simulink model "TST_PTODi_TrqLeadCoord"  (R2016b)
settings: Solver=FixedStepDiscrete  StartTime=0.0  StopTime=simTime  FixedStep=sampleTime  RelTol=1e-3
values from neighbouring files (symbols this model uses):
  testCase = 1    [initTST_PTODi_TrqLeadCoord_001.m]
libraries: simulink x4, UnitTest_Lib x2
settings Model: Creator=zhengjinyan  LastModifiedBy=zhengjinyan
settings DebuggingCC: SignalRangeChecking=error

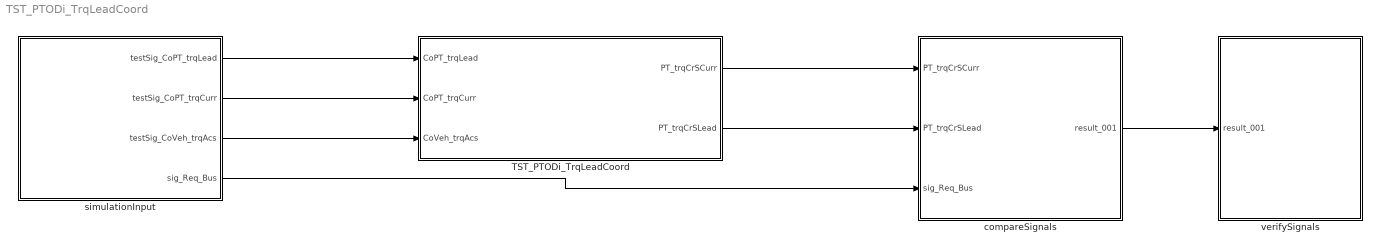
== system TST_PTODi_TrqLeadCoord ==
  TST_PTODi_TrqLeadCoord : Subsystem
  compareSignals : Subsystem
  simulationInput : Subsystem
  verifySignals : Subsystem
  wires:
  simulationInput/1(testSig_CoPT_trqLead) -> TST_PTODi_TrqLeadCoord/1(CoPT_trqLead)
  simulationInput/2(testSig_CoPT_trqCurr) -> TST_PTODi_TrqLeadCoord/2(CoPT_trqCurr)
  simulationInput/3(testSig_CoVeh_trqAcs) -> TST_PTODi_TrqLeadCoord/3(CoVeh_trqAcs)
  TST_PTODi_TrqLeadCoord/1(PT_trqCrSCurr) -> compareSignals/1(PT_trqCrSCurr)
  TST_PTODi_TrqLeadCoord/2(PT_trqCrSLead) -> compareSignals/2(PT_trqCrSLead)
  simulationInput/4(sig_Req_Bus) -> compareSignals/3(sig_Req_Bus)
  compareSignals/1(result_001) -> verifySignals/1(result_001)

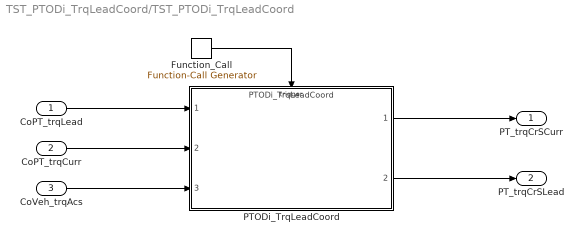
== system TST_PTODi_TrqLeadCoord/TST_PTODi_TrqLeadCoord ==
  CoPT_trqLead : Inport
  CoPT_trqCurr : Inport  Port=2
  CoVeh_trqAcs : Inport  Port=3
  Function_Call : simulink/Ports & Subsystems/Function-Call Generator  sample_time=sampleTime  numberOfIterations=1
  PTODi_TrqLeadCoord : ModelReference  ModelNameDialog=PTODi_TrqLeadCoord  SimulationMode=Normal  ModelReferenceVersion=1.4  TriggerPortName=function  TriggerPortTriggerType=function-call  TriggerPortStatesWhenEnabling=held
  PT_trqCrSCurr : Outport
  PT_trqCrSLead : Outport  Port=2
  wires:
  Function_Call/1 -> PTODi_TrqLeadCoord/Trigger
  CoPT_trqLead/1 -> PTODi_TrqLeadCoord/1
  CoPT_trqCurr/1 -> PTODi_TrqLeadCoord/2
  CoVeh_trqAcs/1 -> PTODi_TrqLeadCoord/3
  PTODi_TrqLeadCoord/1 -> PT_trqCrSCurr/1
  PTODi_TrqLeadCoord/2 -> PT_trqCrSLead/1

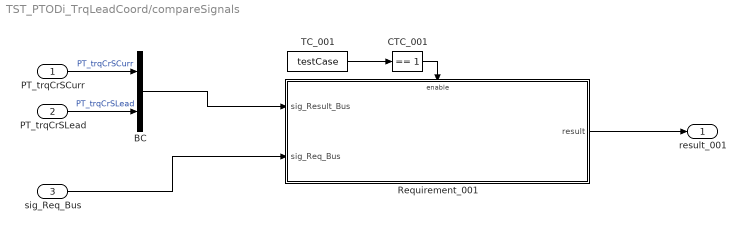
== system TST_PTODi_TrqLeadCoord/compareSignals ==
  PT_trqCrSCurr : Inport
  PT_trqCrSLead : Inport  Port=2
  sig_Req_Bus : Inport  Port=3
  BC : BusCreator  Inputs=2
  CTC_001 : simulink/Logic and Bit Operations/Compare To Constant  relop===  const=1  OutDataTypeStr=boolean
  Requirement_001 : Subsystem
  TC_001 : Constant  Value=testCase
  result_001 : Outport
  wires:
  PT_trqCrSCurr/1 -> BC/1  "PT_trqCrSCurr"
  PT_trqCrSLead/1 -> BC/2  "PT_trqCrSLead"
  TC_001/1 -> CTC_001/1
  CTC_001/1 -> Requirement_001/Enable
  sig_Req_Bus/1 -> Requirement_001/2(sig_Req_Bus)
  BC/1 -> Requirement_001/1(sig_Result_Bus)
  Requirement_001/1(result) -> result_001/1

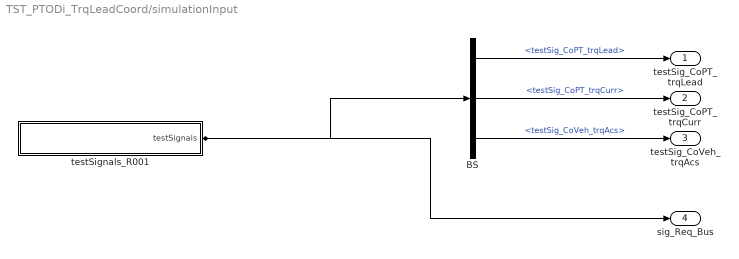
== system TST_PTODi_TrqLeadCoord/simulationInput ==
  BS : BusSelector  OutputSignals=testSig_CoPT_trqLead,testSig_CoPT_trqCurr,testSig_CoVeh_trqAcs
  testSignals_R001 : Subsystem
  testSig_CoPT_trqLead : Outport
  testSig_CoPT_trqCurr : Outport  Port=2
  testSig_CoVeh_trqAcs : Outport  Port=3
  sig_Req_Bus : Outport  Port=4
  wires:
  BS/1 -> testSig_CoPT_trqLead/1  "<testSig_CoPT_trqLead>"
  BS/2 -> testSig_CoPT_trqCurr/1  "<testSig_CoPT_trqCurr>"
  BS/3 -> testSig_CoVeh_trqAcs/1  "<testSig_CoVeh_trqAcs>"
  testSignals_R001/1(testSignals) -> BS/1, sig_Req_Bus/1

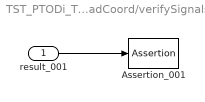
== system TST_PTODi_TrqLeadCoord/verifySignals ==
  result_001 : Inport
  Assertion_001 : Assertion  Enabled=off
  wires:
  result_001/1 -> Assertion_001/1

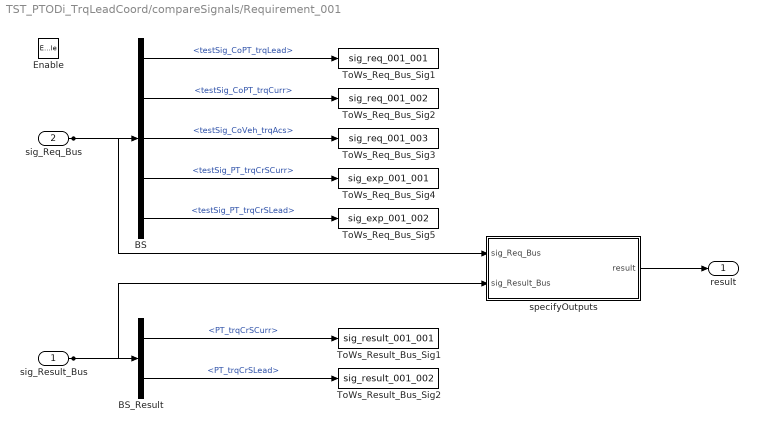
== system TST_PTODi_TrqLeadCoord/compareSignals/Requirement_001 ==
  sig_Result_Bus : Inport
  sig_Req_Bus : Inport  Port=2
  Enable : EnablePort
  BS : BusSelector  OutputSignals=testSig_CoPT_trqLead,testSig_CoPT_trqCurr,testSig_CoVeh_trqAcs,testSig_PT_trqCrSCurr,testSig_PT_trqCrSLead
  BS_Result : BusSelector  OutputSignals=PT_trqCrSCurr,PT_trqCrSLead
  ToWs_Req_Bus_Sig1 : ToWorkspace  VariableName=sig_req_001_001  SaveFormat=Structure With Time
  ToWs_Req_Bus_Sig2 : ToWorkspace  VariableName=sig_req_001_002  SaveFormat=Structure With Time
  ToWs_Req_Bus_Sig3 : ToWorkspace  VariableName=sig_req_001_003  SaveFormat=Structure With Time
  ToWs_Req_Bus_Sig4 : ToWorkspace  VariableName=sig_exp_001_001  SaveFormat=Structure With Time
  ToWs_Req_Bus_Sig5 : ToWorkspace  VariableName=sig_exp_001_002  SaveFormat=Structure With Time
  ToWs_Result_Bus_Sig1 : ToWorkspace  VariableName=sig_result_001_001  SaveFormat=Structure With Time
  ToWs_Result_Bus_Sig2 : ToWorkspace  VariableName=sig_result_001_002  SaveFormat=Structure With Time
  specifyOutputs : Subsystem
  result : Outport
  wires:
  sig_Req_Bus/1 -> BS/1, specifyOutputs/1(sig_Req_Bus)
  BS/1 -> ToWs_Req_Bus_Sig1/1  "<testSig_CoPT_trqLead>"
  BS/2 -> ToWs_Req_Bus_Sig2/1  "<testSig_CoPT_trqCurr>"
  BS/3 -> ToWs_Req_Bus_Sig3/1  "<testSig_CoVeh_trqAcs>"
  BS/4 -> ToWs_Req_Bus_Sig4/1  "<testSig_PT_trqCrSCurr>"
  BS/5 -> ToWs_Req_Bus_Sig5/1  "<testSig_PT_trqCrSLead>"
  sig_Result_Bus/1 -> BS_Result/1, specifyOutputs/2(sig_Result_Bus)
  BS_Result/1 -> ToWs_Result_Bus_Sig1/1  "<PT_trqCrSCurr>"
  BS_Result/2 -> ToWs_Result_Bus_Sig2/1  "<PT_trqCrSLead>"
  specifyOutputs/1(result) -> result/1

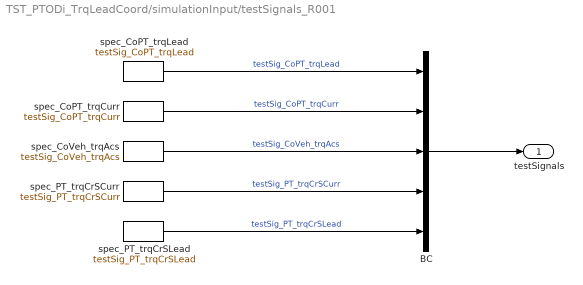
== system TST_PTODi_TrqLeadCoord/simulationInput/testSignals_R001 ==
  BC : BusCreator  Inputs=5
  spec_CoPT_trqCurr : FromWorkspace  VariableName=testSig_CoPT_trqCurr  Interpolate=off  OutputAfterFinalValue=Holding final value
  spec_CoPT_trqLead : FromWorkspace  VariableName=testSig_CoPT_trqLead  Interpolate=off  OutputAfterFinalValue=Holding final value
  spec_CoVeh_trqAcs : FromWorkspace  VariableName=testSig_CoVeh_trqAcs  Interpolate=off  OutputAfterFinalValue=Holding final value
  spec_PT_trqCrSCurr : FromWorkspace  VariableName=testSig_PT_trqCrSCurr  Interpolate=off  OutputAfterFinalValue=Holding final value
  spec_PT_trqCrSLead : FromWorkspace  VariableName=testSig_PT_trqCrSLead  Interpolate=off  OutputAfterFinalValue=Holding final value
  testSignals : Outport
  wires:
  BC/1 -> testSignals/1
  spec_CoPT_trqLead/1 -> BC/1  "testSig_CoPT_trqLead"
  spec_CoPT_trqCurr/1 -> BC/2  "testSig_CoPT_trqCurr"
  spec_CoVeh_trqAcs/1 -> BC/3  "testSig_CoVeh_trqAcs"
  spec_PT_trqCrSCurr/1 -> BC/4  "testSig_PT_trqCrSCurr"
  spec_PT_trqCrSLead/1 -> BC/5  "testSig_PT_trqCrSLead"

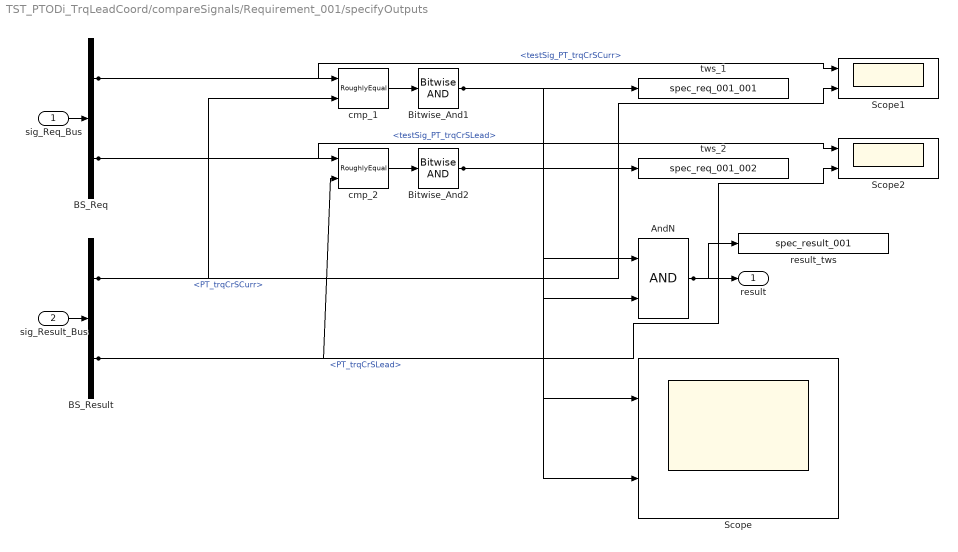
== system TST_PTODi_TrqLeadCoord/compareSignals/Requirement_001/specifyOutputs ==
  sig_Req_Bus : Inport
  sig_Result_Bus : Inport  Port=2
  AndN : Logic
  BS_Req : BusSelector  OutputSignals=testSig_PT_trqCrSCurr,testSig_PT_trqCrSLead
  BS_Result : BusSelector  OutputSignals=PT_trqCrSCurr,PT_trqCrSLead
  Bitwise_And1 : simulink/Logic and Bit Operations/Bitwise Operator  logicop=AND  UseBitMask=off  BitMask=bin2dec('11011001')  BitMaskRealWorld=Stored Integer
  Bitwise_And2 : simulink/Logic and Bit Operations/Bitwise Operator  logicop=AND  UseBitMask=off  BitMask=bin2dec('11011001')  BitMaskRealWorld=Stored Integer
  Scope : Scope  NumInputPorts=2
  Scope1 : Scope  NumInputPorts=2
  Scope2 : Scope  NumInputPorts=2
  cmp_1 : UnitTest_Lib/RoughlyEqual  slope=0.1
  cmp_2 : UnitTest_Lib/RoughlyEqual  slope=0.1
  result_tws : ToWorkspace  VariableName=spec_result_001
  tws_1 : ToWorkspace  VariableName=spec_req_001_001
  tws_2 : ToWorkspace  VariableName=spec_req_001_002
  result : Outport
  wires:
  sig_Req_Bus/1 -> BS_Req/1
  sig_Result_Bus/1 -> BS_Result/1
  AndN/1 -> result/1, result_tws/1
  BS_Req/1 -> cmp_1/1, Scope1/1  "<testSig_PT_trqCrSCurr>"
  BS_Result/1 -> cmp_1/2, Scope1/2  "<PT_trqCrSCurr>"
  cmp_1/1 -> Bitwise_And1/1
  Bitwise_And1/1 -> tws_1/1, AndN/1, Scope/1
  BS_Req/2 -> cmp_2/1, Scope2/1  "<testSig_PT_trqCrSLead>"
  BS_Result/2 -> cmp_2/2, Scope2/2  "<PT_trqCrSLead>"
  cmp_2/1 -> Bitwise_And2/1
  Bitwise_And2/1 -> tws_2/1, AndN/2, Scope/2
